simulink model "xb_fft_32pt_core"  (Simulink 7.8)
settings: Solver=ode45  StartTime=0.0  StopTime=10.0  RelTol=1e-3
libraries: xbsIndex_r4 x1517, xbsReplacements_r4 x12
(part 1 of 9)
settings Model: Creator=dan  LastModifiedBy=dan
settings DebuggingCC: FcnCallInpInsideContextMsg=Use local settings  StrictBusMsg=Warning

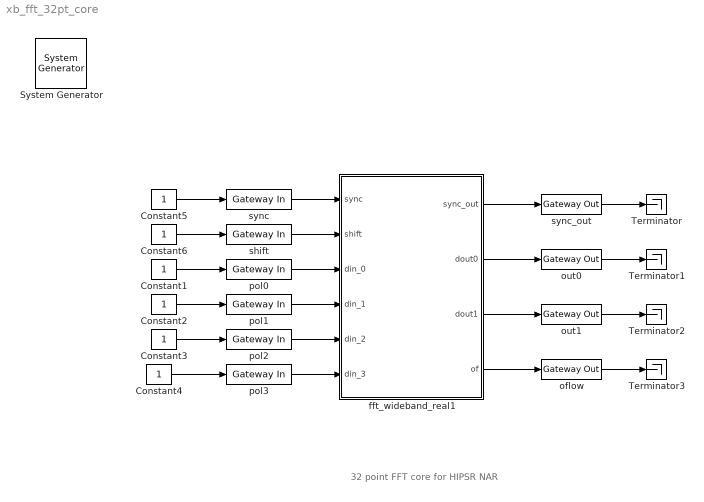
== system xb_fft_32pt_core ==
  note: 32 point FFT core for HIPSR NAR
  " System Generator" : xbsIndex_r4/ System Generator  Tag=genX  xilinxfamily=virtex5  part=xc5vsx95t  speed=-2  package=ff1136  synthesis_tool=XST  clock_wrapper=Clock Enables  directory=/designs/dan/13.x/designs/old/noise_diode/bb/xb_fft_32pt_core  proj_type=Project Navigator  Synth_file=XST Defaults  Impl_file=ISE Defaults  testbench=off  simulink_period=1  sysclk_period=10  dcm_input_clock_period=10  incr_netlist=off  trim_vbits=Everywhere in SubSystem  dbl_ovrd=According to Block Masks  core_generation=According to Block Masks  run_coregen=off  deprecated_control=off  eval_field=0  block_type=sysgen
      settings: block_version=11.4
  Constant{1..6} (6 alike) : Constant
  Terminator{,1..3} (4 alike) : Terminator
  fft_wideband_real1 : Subsystem  AncestorBlock=xblocks_library_ffts/fft_wideband_real  mask(fft_wideband_real){FFTSize=5, n_inputs=2, input_bit_width=18, coeff_bit_width=18, unscramble=on, add_latency=2, mult_latency=3, bram_latency=2, conv_latency=1, input_latency=0, biplex_direct_latency=0, quantization=Truncate, overflow=Wrap, arch=Virtex5, opt_target=logic, coeffs_bit_limit=11, delays_bit_limit=11, specify_mult=on, mult_spec=ones(1,5), hardcode_shifts=on, shift_schedule=ones(1,5), dsp48_adders=on, bit_growth_chart=[0], negate_latency=3, negate_dsp48e=on}
      mask prompts: FFTSize "Size of FFT: (2^? pts)"; n_inputs "Number of Simultaneous Inputs: (2^?)"; input_bit_width "Input Bit Width"; coeff_bit_width "Coefficient Bit Width"; unscramble "Unscramble output (ie, put channels in canonical order)"; add_latency "Add Latency"; mult_latency "Mult Latency"; bram_latency "BRAM Latency"; conv_latency "Convert Latency"; input_latency "Input Latency"; biplex_direct_latency "Latency between biplexes and fft_direct"; quantization "Quantization Behavior"; overflow "Overflow Behavior"; arch "Architecture"; opt_target "Use less"; coeffs_bit_limit "Number bits above which to store stage's coefficients in BRAM (2^? bits)"; delays_bit_limit "Number bits above which to store stage's delays in BRAM (2^? bits)"; specify_mult "Specify multiplier use (behavioral HDL if not specified)"; mult_spec "Multiplier specification (0=core, 1=embedded, 2=behavioural) (left=1st stage)"; hardcode_shifts "Hardcode shift schedule"; shift_schedule "Shift schedule"; dsp48_adders "DSP48 adders in butterfly"; bit_growth_chart "Bit growth vector"; negate_latency "Negate latency"; negate_dsp48e "Negate with DSP48E"
      mask help:
      | A real-sampled wideband FFT.
      |
      | (xBlock version)
      mask init:
      | config.source = str2func('fft_wideband_real_init_xblock');
      | config.toplevel = gcb;
      | config.depend = get_dependlist('fft_wideband_real');
      | set_param(gcb,'LinkStatus','inactive');
      | xBlock(config, {config.toplevel, ...
      |    'FFTSize', FFTSize, ...
      |    'n_inputs', n_inputs, ...
      |    'input_bit_width', input_bit_width, ...
      |    'coeff_bit_width', coeff_bit_width, ...
      |    'unscramble', unscramble, ...
      |    'add_latency', add_latency, ...
      |    'mult_latency', mult_latency, ...
      |    'bram_latency', bram_latency, ...
      |    'conv_latency', conv_latency, ...
      |    'input_latency', input_latency, ...
      |    'biplex_direct_latency', biplex_direct_latency, ...
      |    'quantization', quantization, ...
      |    'overflow', overflow, ...
      |    'arch', arch, ...
      |    'opt_target', opt_target, ...
      |    'coeffs_bit_limit', coeffs_bit_limit, ...
      |    'delays_bit_limit', delays_bit_limit, ...    
      |    'specify_mult', specify_mult, ...
      |    'mult_spec', mult_spec, ...
      |    'hardcode_shifts', hardcode_shifts, ...
      |    'shift_schedule', shift_schedule, ...
      |    'dsp48_adders', dsp48_adders, ...
      |    'bit_growth_chart', bit_growth_chart, ....
      |    'negate_latency', negate_latency, ...
      |    'negate_dsp48e', negate_dsp48e, ...
      | });
      settings: CopyFcn=fft_wideband_real_init(gcb);
      settings: AttributesFormatString=|
      | 5 stages
      | (18,18)
      | Truncate
      | Wrap
      | 0 0 0 0 0 0
      mask Help: eval('xlWeb(''http://casper.berkeley.edu/wiki/Fft_wideband_real'')')
      mask StyleString: edit,edit,edit,edit,checkbox,edit,edit,edit,edit,edit,edit,popup(Truncate|Round  (unbiased: +/- Inf)|Round  (unbiased: Even Values)),popup(Wrap|Saturate|Error),popup(Virtex2Pro|Virtex5),popup(logic|multipliers),edit,edit,checkbox,edit,checkbox,edit,checkbox,edit,edit,checkbox
      mask CallbackString:
      | bit_growth_chart = eval(get_param(gcb,'bit_growth_chart'));
      | FFTSize = eval(get_param(gcb,'FFTSize'));
      | bit_growth_chart = [reshape(bit_growth_chart, 1, []) zeros(1,FFTSize)];
      | bit_growth_sum = sum(bit_growth_chart(1:FFTSize));
      | input_bit_width = eval(get_param(gcb,'input_bit_width'));
      | if input_bit_width + bit_growth_sum > 18
      |     disp('Total bit width cannot exceed 18. Forcing to 0 bit growth');
      |     set_param(gcb,'bit_growth_chart','[0]');
      | end||bit_growth_chart = eval(get_param(gcb,'bit_growth_chart'));
      | FFTSize = eval(get_param(gcb,'FFTSize'));
      | bit_growth_chart = [reshape(bit_growth_chart, 1, []) zeros(1,FFTSize)];
      | bit_growth_sum = sum(bit_growth_chart(1:FFTSize));
      | input_bit_width = eval(get_param(gcb,'input_bit_width'));
      | if input_bit_width + bit_growth_sum > 18
      |     disp('Total bit width cannot exceed 18. Forcing to 0 bit growth');
      |     set_param(gcb,'bit_growth_chart','[0]');
      | end|||||||||||fft_callback_arch(gcb);||||specify_mult = get_param(gcb, 'specify_mult');
      | set_param_state(gcb, 'mult_spec', specify_mult);||hardcode_shifts = get_param(gcb, 'hardcode_shifts');
      | set_param_state(gcb, 'shift_schedule', hardcode_shifts);||fft_callback_dsp48_adders(gcb);|bit_growth_chart = eval(get_param(gcb,'bit_growth_chart'));
      | FFTSize = eval(get_param(gcb,'FFTSize'));
      | bit_growth_chart = [reshape(bit_growth_chart, 1, []) zeros(1,FFTSize)];
      | bit_growth_sum = sum(bit_growth_chart(1:FFTSize));
      | input_bit_width = eval(get_param(gcb,'input_bit_width'));
      | if input_bit_width + bit_growth_sum > 18
      |     disp('Total bit width cannot exceed 18. Forcing to 0 bit growth');
      |     set_param(gcb,'bit_growth_chart','[0]');
      | end||
      mask TabNameString: Basic,Basic,Basic,Basic,Basic,Latency,Latency,Latency,Latency,Latency,Latency,Implementation,Implementation,Implementation,Implementation,Implementation,Implementation,Implementation,Implementation,Implementation,Implementation,Implementation,Basic,Basic,Basic
  oflow : xbsIndex_r4/Gateway Out  inherit_from_input=off  hdl_port=on  timing_constraint=None  locs_specified=off  LOCs={}  UseAsDAC=off  DACChannel='1'  block_type=gatewayout
      settings: infoedit="Gateway out block.  Converts Xilinx fixed point inputs into ouputs of type Simulink integer, double, or fixed point.<br><br>Hardware notes:  In hardware these blocks become top level output ports or are discarded, depending on how they are configured."  block_version=11.4
  out0 : xbsIndex_r4/Gateway Out  inherit_from_input=off  hdl_port=on  timing_constraint=None  locs_specified=off  LOCs={}  UseAsDAC=off  DACChannel='1'  block_type=gatewayout
      settings: infoedit="Gateway out block.  Converts Xilinx fixed point inputs into ouputs of type Simulink integer, double, or fixed point.<br><br>Hardware notes:  In hardware these blocks become top level output ports or are discarded, depending on how they are configured."  block_version=11.4
  out1 : xbsIndex_r4/Gateway Out  inherit_from_input=off  hdl_port=on  timing_constraint=None  locs_specified=off  LOCs={}  UseAsDAC=off  DACChannel='1'  block_type=gatewayout
      settings: infoedit="Gateway out block.  Converts Xilinx fixed point inputs into ouputs of type Simulink integer, double, or fixed point.<br><br>Hardware notes:  In hardware these blocks become top level output ports or are discarded, depending on how they are configured."  block_version=11.4
  pol{0..3} (4 alike) : xbsIndex_r4/Gateway In  gui_display_data_type=Fixed-point  arith_type="Signed  (2's comp)"  n_bits=18  bin_pt=17  preci_type=Single  exp_width=8  frac_width=24  quantization="Round  (unbiased: +/- Inf)"  overflow=Saturate  period=1  dbl_ovrd=off  timing_constraint=None  locs_specified=off  LOCs={}  inherit_from_input=off  UseAsADC=off  ADCChannel='1'  hdl_port=on  block_type=gatewayin
      settings: infoedit="Gateway in block.  Converts inputs of type Simulink integer, double and fixed point to  Xilinx fixed point type.<br><br>Hardware notes:  In hardware these blocks become top level input ports."  block_version=11.4
  shift : xbsIndex_r4/Gateway In  gui_display_data_type=Fixed-point  arith_type=Unsigned  n_bits=32  bin_pt=0  preci_type=Single  exp_width=8  frac_width=24  quantization="Round  (unbiased: +/- Inf)"  overflow=Saturate  period=1  dbl_ovrd=off  timing_constraint=None  locs_specified=off  LOCs={}  inherit_from_input=off  UseAsADC=off  ADCChannel='1'  hdl_port=on  block_type=gatewayin
      settings: infoedit="Gateway in block.  Converts inputs of type Simulink integer, double and fixed point to  Xilinx fixed point type.<br><br>Hardware notes:  In hardware these blocks become top level input ports."  block_version=11.4
  sync : xbsIndex_r4/Gateway In  gui_display_data_type=Fixed-point  arith_type=Boolean  n_bits=16  bin_pt=14  preci_type=Single  exp_width=8  frac_width=24  quantization="Round  (unbiased: +/- Inf)"  overflow=Saturate  period=1  dbl_ovrd=off  timing_constraint=None  locs_specified=off  LOCs={}  inherit_from_input=off  UseAsADC=off  ADCChannel='1'  hdl_port=on  block_type=gatewayin
      settings: infoedit="Gateway in block.  Converts inputs of type Simulink integer, double and fixed point to  Xilinx fixed point type.<br><br>Hardware notes:  In hardware these blocks become top level input ports."  block_version=11.4
  sync_out : xbsIndex_r4/Gateway Out  inherit_from_input=off  hdl_port=on  timing_constraint=None  locs_specified=off  LOCs={}  UseAsDAC=off  DACChannel='1'  block_type=gatewayout
      settings: infoedit="Gateway out block.  Converts Xilinx fixed point inputs into ouputs of type Simulink integer, double, or fixed point.<br><br>Hardware notes:  In hardware these blocks become top level output ports or are discarded, depending on how they are configured."  block_version=11.4
  wires:
  Constant5/1 -> sync/1
  Constant1/1 -> pol0/1
  Constant4/1 -> pol3/1
  Constant3/1 -> pol2/1
  Constant2/1 -> pol1/1
  Constant6/1 -> shift/1
  fft_wideband_real1/1(sync_out) -> sync_out/1
  fft_wideband_real1/2(dout0) -> out0/1
  fft_wideband_real1/3(dout1) -> out1/1
  fft_wideband_real1/4(of) -> oflow/1
  sync_out/1 -> Terminator/1
  oflow/1 -> Terminator3/1
  out1/1 -> Terminator2/1
  out0/1 -> Terminator1/1
  sync/1 -> fft_wideband_real1/1(sync)
  shift/1 -> fft_wideband_real1/2(shift)
  pol0/1 -> fft_wideband_real1/3(din_0)
  pol1/1 -> fft_wideband_real1/4(din_1)
  pol2/1 -> fft_wideband_real1/5(din_2)
  pol3/1 -> fft_wideband_real1/6(din_3)

== system xb_fft_32pt_core/fft_wideband_real1 ==
  sync : Inport
  shift : Inport  Port=2
  din_0 : Inport  Port=3
  din_1 : Inport  Port=4
  din_2 : Inport  Port=5
  din_3 : Inport  Port=6
  fft_biplex_real_4x0 : Subsystem
      settings: AttributesFormatString=|
      | Virtex5
      | 3 stages
      | [18,18]
      | Truncate
      | Wrap
      | 0 0 0 0 0 0 0 0 0
  fft_direct : Subsystem
      settings: AttributesFormatString=|
      | Virtex5
      | stages [4  5] of 5
      | [18,18]
      | Truncate
      | Wrap
      | 0 0 0 0 0
  fft_unscrambler : Subsystem
      settings: AttributesFormatString=FFTSize=4, n_inputs=1
  in_del_4x0pol1 : Subsystem
      settings: AttributesFormatString=Latency = 0
  in_del_4x0pol2 : Subsystem
      settings: AttributesFormatString=Latency = 0
  in_del_4x0pol3 : Subsystem
      settings: AttributesFormatString=Latency = 0
  in_del_4x0pol4 : Subsystem
      settings: AttributesFormatString=Latency = 0
  in_del_sync_4x0 : Subsystem
      settings: AttributesFormatString=Latency = 0
  of_det : xbsIndex_r4/Logical  logical_function=OR  inputs=2  en=off  latency=1  precision=Full  arith_type=Unsigned  n_bits=16  bin_pt=0  align_bp=on  dbl_ovrd=off  block_type=logical
  out_del_4x0pol1 : Subsystem
      settings: AttributesFormatString=Latency = 0
  out_del_4x0pol2 : Subsystem
      settings: AttributesFormatString=Latency = 0
  out_del_4x0pol3 : Subsystem
      settings: AttributesFormatString=Latency = 0
  out_del_4x0pol4 : Subsystem
      settings: AttributesFormatString=Latency = 0
  out_del_sync_4x0 : Subsystem
      settings: AttributesFormatString=Latency = 0
  shift_slice : xbsIndex_r4/Slice  nbits=2  boolean_output=off  mode=Lower Bit Location + Width  bit1=0  base1=MSB of Input  bit0=3  base0=LSB of Input  dbl_ovrd=off  block_type=slice
  sync_out : Outport
  dout0 : Outport  Port=2
  dout1 : Outport  Port=3
  of : Outport  Port=4
  wires:
  shift/1 -> fft_biplex_real_4x0/2(shift), shift_slice/1
  of_det/1 -> of/1
  fft_direct/6(of) -> of_det/2
  fft_biplex_real_4x0/6(of) -> of_det/1
  fft_unscrambler/3(Out2) -> dout1/1
  fft_unscrambler/2(Out1) -> dout0/1
  fft_unscrambler/1(sync_out) -> sync_out/1
  fft_direct/3(dout_1) -> fft_unscrambler/3(In2)
  fft_direct/2(dout_0) -> fft_unscrambler/2(In1)
  fft_direct/1(sync_out) -> fft_unscrambler/1(sync)
  out_del_4x0pol4/1(q) -> fft_direct/6(din_3)
  out_del_4x0pol3/1(q) -> fft_direct/5(din_2)
  out_del_4x0pol2/1(q) -> fft_direct/4(din_1)
  out_del_4x0pol1/1(q) -> fft_direct/3(din_0)
  shift_slice/1 -> fft_direct/2(shift)
  out_del_sync_4x0/1(q) -> fft_direct/1(sync)
  fft_biplex_real_4x0/1(sync_out) -> out_del_sync_4x0/1(d)
  fft_biplex_real_4x0/5(pol4_out) -> out_del_4x0pol4/1(d)
  fft_biplex_real_4x0/4(pol3_out) -> out_del_4x0pol3/1(d)
  fft_biplex_real_4x0/3(pol2_out) -> out_del_4x0pol2/1(d)
  fft_biplex_real_4x0/2(pol1_out) -> out_del_4x0pol1/1(d)
  in_del_4x0pol4/1(q) -> fft_biplex_real_4x0/6(pol4)
  in_del_4x0pol3/1(q) -> fft_biplex_real_4x0/5(pol3)
  in_del_4x0pol2/1(q) -> fft_biplex_real_4x0/4(pol2)
  in_del_4x0pol1/1(q) -> fft_biplex_real_4x0/3(pol1)
  in_del_sync_4x0/1(q) -> fft_biplex_real_4x0/1(sync)
  din_3/1 -> in_del_4x0pol4/1(d)
  din_2/1 -> in_del_4x0pol3/1(d)
  din_1/1 -> in_del_4x0pol2/1(d)
  din_0/1 -> in_del_4x0pol1/1(d)
  sync/1 -> in_del_sync_4x0/1(d)

== system xb_fft_32pt_core/fft_wideband_real1/fft_biplex_real_4x0 ==
  sync : Inport
  shift : Inport  Port=2
  pol1 : Inport  Port=3
  pol2 : Inport  Port=4
  pol3 : Inport  Port=5
  pol4 : Inport  Port=6
  bi_real_unscr_4x : Subsystem
  biplex_core : Subsystem
      settings: AttributesFormatString=|
      | 3 stages
      | reduce logic
      | Virtex5
  ri_to_c_pol1 : Subsystem
  ri_to_c_pol2 : Subsystem
  sync_out : Outport
  pol1_out : Outport  Port=2
  pol2_out : Outport  Port=3
  pol3_out : Outport  Port=4
  pol4_out : Outport  Port=5
  of : Outport  Port=6
  wires:
  bi_real_unscr_4x/5(pol4_out) -> pol4_out/1
  bi_real_unscr_4x/4(pol3_out) -> pol3_out/1
  bi_real_unscr_4x/3(pol2_out) -> pol2_out/1
  bi_real_unscr_4x/2(pol1_out) -> pol1_out/1
  bi_real_unscr_4x/1(sync_out) -> sync_out/1
  biplex_core/3(out2) -> bi_real_unscr_4x/3(odd)
  biplex_core/2(out1) -> bi_real_unscr_4x/2(even)
  biplex_core/1(sync_out) -> bi_real_unscr_4x/1(sync)
  biplex_core/4(of) -> of/1
  ri_to_c_pol2/1(c) -> biplex_core/4(pol2)
  ri_to_c_pol1/1(c) -> biplex_core/3(pol1)
  shift/1 -> biplex_core/2(shift)
  sync/1 -> biplex_core/1(sync)
  pol4/1 -> ri_to_c_pol2/2(im)
  pol3/1 -> ri_to_c_pol2/1(re)
  pol2/1 -> ri_to_c_pol1/2(im)
  pol1/1 -> ri_to_c_pol1/1(re)

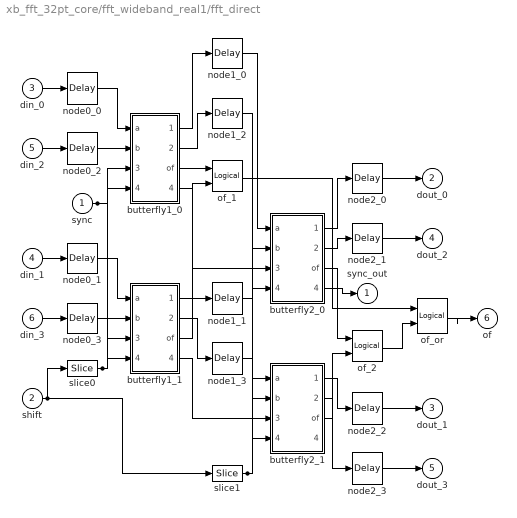
== system xb_fft_32pt_core/fft_wideband_real1/fft_direct ==
  sync : Inport
  shift : Inport  Port=2
  din_0 : Inport  Port=3
  din_1 : Inport  Port=4
  din_2 : Inport  Port=5
  din_3 : Inport  Port=6
  butterfly1_0 : Subsystem
      settings: AttributesFormatString=|
      | twiddle_general_4mult
      | coeffs in slices
      | Bit growth:0
  butterfly1_1 : Subsystem
      settings: AttributesFormatString=|
      | twiddle_general_4mult
      | coeffs in slices
      | Bit growth:0
  butterfly2_0 : Subsystem
      settings: AttributesFormatString=|
      | twiddle_general_4mult
      | coeffs in slices
      | Bit growth:0
  butterfly2_1 : Subsystem
      settings: AttributesFormatString=|
      | twiddle_general_4mult
      | coeffs in slices
      | Bit growth:0
  node0_{0..3} (4 alike) : xbsIndex_r4/Delay  rst=off  infoeditControl=Selection of Reset will increase slice count due to use of real FFs and instead of SRLs  en=off  latency=0  dbl_ovrd=off  reg_retiming=off  block_type=delay
  node1_{0..3} (4 alike) : xbsIndex_r4/Delay  rst=off  infoeditControl=Selection of Reset will increase slice count due to use of real FFs and instead of SRLs  en=off  latency=0  dbl_ovrd=off  reg_retiming=off  block_type=delay
  node2_{0..3} (4 alike) : xbsIndex_r4/Delay  rst=off  infoeditControl=Selection of Reset will increase slice count due to use of real FFs and instead of SRLs  en=off  latency=0  dbl_ovrd=off  reg_retiming=off  block_type=delay
  of_1 : xbsIndex_r4/Logical  logical_function=OR  inputs=2  en=off  latency=1  precision=Full  arith_type=Unsigned  n_bits=16  bin_pt=0  align_bp=on  dbl_ovrd=off  block_type=logical
  of_2 : xbsIndex_r4/Logical  logical_function=OR  inputs=2  en=off  latency=1  precision=Full  arith_type=Unsigned  n_bits=16  bin_pt=0  align_bp=on  dbl_ovrd=off  block_type=logical
  of_or : xbsIndex_r4/Logical  logical_function=OR  inputs=2  en=off  latency=0  precision=Full  arith_type=Unsigned  n_bits=16  bin_pt=0  align_bp=on  dbl_ovrd=off  block_type=logical
  slice0 : xbsIndex_r4/Slice  nbits=1  boolean_output=on  mode=Lower Bit Location + Width  bit1=0  base1=MSB of Input  bit0=0  base0=LSB of Input  dbl_ovrd=off  block_type=slice
  slice1 : xbsIndex_r4/Slice  nbits=1  boolean_output=on  mode=Lower Bit Location + Width  bit1=0  base1=MSB of Input  bit0=1  base0=LSB of Input  dbl_ovrd=off  block_type=slice
  sync_out : Outport
  dout_0 : Outport  Port=2
  dout_1 : Outport  Port=3
  dout_2 : Outport  Port=4
  dout_3 : Outport  Port=5
  of : Outport  Port=6
  wires:
  shift/1 -> slice1/1, slice0/1
  sync/1 -> butterfly1_1/3(sync), butterfly1_0/3(sync)
  slice0/1 -> butterfly1_1/4(shift), butterfly1_0/4(shift)
  slice1/1 -> butterfly2_1/4(shift), butterfly2_0/4(shift)
  butterfly2_0/4(sync_out) -> sync_out/1
  of_or/1 -> of/1
  of_2/1 -> of_or/2
  of_1/1 -> of_or/1
  butterfly2_1/3(of) -> of_2/2
  butterfly2_0/3(of) -> of_2/1
  butterfly2_1/2(a-bw) -> node2_3/1
  butterfly2_1/1(a+bw) -> node2_2/1
  butterfly1_1/4(sync_out) -> butterfly2_1/3(sync)
  node1_3/1 -> butterfly2_1/2(b)
  node1_2/1 -> butterfly2_1/1(a)
  butterfly2_0/2(a-bw) -> node2_1/1
  butterfly2_0/1(a+bw) -> node2_0/1
  butterfly1_0/4(sync_out) -> butterfly2_0/3(sync)
  node1_1/1 -> butterfly2_0/2(b)
  node1_0/1 -> butterfly2_0/1(a)
  butterfly1_1/3(of) -> of_1/2
  butterfly1_0/3(of) -> of_1/1
  butterfly1_1/2(a-bw) -> node1_3/1
  butterfly1_1/1(a+bw) -> node1_1/1
  node0_3/1 -> butterfly1_1/2(b)
  node0_1/1 -> butterfly1_1/1(a)
  butterfly1_0/2(a-bw) -> node1_2/1
  butterfly1_0/1(a+bw) -> node1_0/1
  node0_2/1 -> butterfly1_0/2(b)
  node0_0/1 -> butterfly1_0/1(a)
  node2_3/1 -> dout_3/1
  node2_2/1 -> dout_1/1
  node2_1/1 -> dout_2/1
  node2_0/1 -> dout_0/1
  din_3/1 -> node0_3/1
  din_2/1 -> node0_2/1
  din_1/1 -> node0_1/1
  din_0/1 -> node0_0/1

== system xb_fft_32pt_core/fft_wideband_real1/fft_unscrambler ==
  sync : Inport
  In1 : Inport  Port=2
  In2 : Inport  Port=3
  const : xbsIndex_r4/Constant  const=1  gui_display_data_type=Fixed-point  arith_type=Boolean  n_bits=1  bin_pt=0  preci_type=Single  exp_width=8  frac_width=24  explicit_period=on  period=1  equ=P=C  opselect=C  inp2=PCIN>>17  opr=+  inp1=P  carry=CIN  dbl_ovrd=off  block_type=constant
  reorder1 : Subsystem
      settings: AttributesFormatString=order=3
  square_transposer1 : Subsystem
      settings: AttributesFormatString=n_inputs=1
  sync_out : Outport
  Out1 : Outport  Port=2
  Out2 : Outport  Port=3
  wires:
  square_transposer1/3(Out2) -> reorder1/4(din1)  "xlsub2_reorder_In2"
  square_transposer1/2(Out1) -> reorder1/3(din0)  "xlsub2_reorder_In1"
  square_transposer1/1(sync_out) -> reorder1/1(sync)
  In2/1 -> square_transposer1/3(In2)
  In1/1 -> square_transposer1/2(In1)
  sync/1 -> square_transposer1/1(sync)
  reorder1/4(dout1) -> Out2/1
  reorder1/3(dout0) -> Out1/1
  reorder1/1(sync_out) -> sync_out/1
  const/1 -> reorder1/2(en)

== system xb_fft_32pt_core/fft_wideband_real1/in_del_4x0pol1 ==
  d : Inport
  q : Outport
  wires:
  d/1 -> q/1

== system xb_fft_32pt_core/fft_wideband_real1/in_del_4x0pol2 ==
  d : Inport
  q : Outport
  wires:
  d/1 -> q/1

== system xb_fft_32pt_core/fft_wideband_real1/in_del_4x0pol3 ==
  d : Inport
  q : Outport
  wires:
  d/1 -> q/1

== system xb_fft_32pt_core/fft_wideband_real1/in_del_4x0pol4 ==
  d : Inport
  q : Outport
  wires:
  d/1 -> q/1

== system xb_fft_32pt_core/fft_wideband_real1/in_del_sync_4x0 ==
  d : Inport
  q : Outport
  wires:
  d/1 -> q/1

== system xb_fft_32pt_core/fft_wideband_real1/out_del_4x0pol1 ==
  d : Inport
  q : Outport
  wires:
  d/1 -> q/1

== system xb_fft_32pt_core/fft_wideband_real1/out_del_4x0pol2 ==
  d : Inport
  q : Outport
  wires:
  d/1 -> q/1

== system xb_fft_32pt_core/fft_wideband_real1/out_del_4x0pol3 ==
  d : Inport
  q : Outport
  wires:
  d/1 -> q/1

== system xb_fft_32pt_core/fft_wideband_real1/out_del_4x0pol4 ==
  d : Inport
  q : Outport
  wires:
  d/1 -> q/1

== system xb_fft_32pt_core/fft_wideband_real1/out_del_sync_4x0 ==
  d : Inport
  q : Outport
  wires:
  d/1 -> q/1

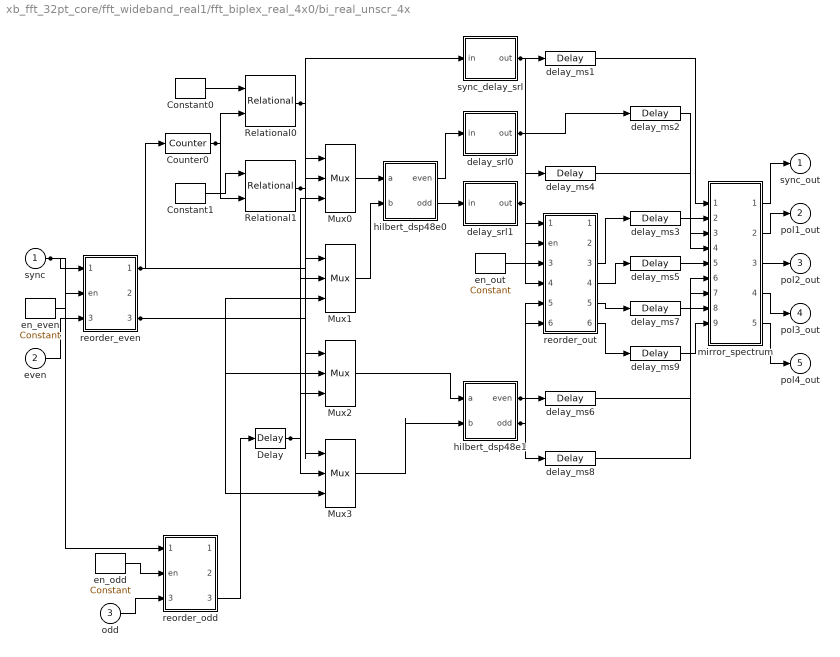
== system xb_fft_32pt_core/fft_wideband_real1/fft_biplex_real_4x0/bi_real_unscr_4x ==
  sync : Inport
  even : Inport  Port=2
  odd : Inport  Port=3
  Constant0 : xbsIndex_r4/Constant  const=3  gui_display_data_type=Fixed-point  arith_type=Unsigned  n_bits=3  bin_pt=0  preci_type=Single  exp_width=8  frac_width=24  explicit_period=on  period=1  equ=P=C  opselect=C  inp2=PCIN>>17  opr=+  inp1=P  carry=CIN  dbl_ovrd=off  block_type=constant
  Constant1 : xbsIndex_r4/Constant  const=7  gui_display_data_type=Fixed-point  arith_type=Unsigned  n_bits=3  bin_pt=0  preci_type=Single  exp_width=8  frac_width=24  explicit_period=on  period=1  equ=P=C  opselect=C  inp2=PCIN>>17  opr=+  inp1=P  carry=CIN  dbl_ovrd=off  block_type=constant
  Counter0 : xbsIndex_r4/Counter  cnt_type=Free Running  cnt_to=Inf  operation=Up  start_count=0  cnt_by_val=1  arith_type=Unsigned  n_bits=3  bin_pt=0  load_pin=off  rst=on  en=off  explicit_period=on  period=1  dbl_ovrd=off  use_behavioral_HDL=off  implementation=Fabric  block_type=counter
  Delay : xbsIndex_r4/Delay  rst=off  infoeditControl=Selection of Reset will increase slice count due to use of real FFs and instead of SRLs  en=off  latency=1  dbl_ovrd=off  reg_retiming=off  block_type=delay
  Mux{0..3} (4 alike) : xbsIndex_r4/Mux  inputs=2  en=off  latency=1  precision=Full  arith_type=Unsigned  n_bits=16  bin_pt=14  quantization=Truncate  overflow=Wrap  dbl_ovrd=off  block_type=mux
  Relational0 : xbsIndex_r4/Relational  mode=a=b  en=off  latency=1  dbl_ovrd=off  block_type=relational
  Relational1 : xbsIndex_r4/Relational  mode=a=b  en=off  latency=1  dbl_ovrd=off  block_type=relational
  delay_ms{1..9} (9 alike) : xbsIndex_r4/Delay  rst=off  infoeditControl=Selection of Reset will increase slice count due to use of real FFs and instead of SRLs  en=off  latency=1  dbl_ovrd=off  reg_retiming=off  block_type=delay
  delay_srl0 : Subsystem
  delay_srl1 : Subsystem
  en_even : xbsIndex_r4/Constant  const=1  gui_display_data_type=Fixed-point  arith_type=Boolean  n_bits=1  bin_pt=0  preci_type=Single  exp_width=8  frac_width=24  explicit_period=on  period=1  equ=P=C  opselect=C  inp2=PCIN>>17  opr=+  inp1=P  carry=CIN  dbl_ovrd=off  block_type=constant
  en_odd : xbsIndex_r4/Constant  const=1  gui_display_data_type=Fixed-point  arith_type=Boolean  n_bits=1  bin_pt=0  preci_type=Single  exp_width=8  frac_width=24  explicit_period=on  period=1  equ=P=C  opselect=C  inp2=PCIN>>17  opr=+  inp1=P  carry=CIN  dbl_ovrd=off  block_type=constant
  en_out : xbsIndex_r4/Constant  const=1  gui_display_data_type=Fixed-point  arith_type=Boolean  n_bits=1  bin_pt=0  preci_type=Single  exp_width=8  frac_width=24  explicit_period=on  period=1  equ=P=C  opselect=C  inp2=PCIN>>17  opr=+  inp1=P  carry=CIN  dbl_ovrd=off  block_type=constant
  hilbert_dsp48e0 : Subsystem
  hilbert_dsp48e1 : Subsystem
  mirror_spectrum : Subsystem
  reorder_even : Subsystem
      settings: AttributesFormatString=order=2
  reorder_odd : Subsystem
      settings: AttributesFormatString=order=2
  reorder_out : Subsystem
      settings: AttributesFormatString=order=2
  sync_delay_srl : Subsystem
  sync_out : Outport
  pol1_out : Outport  Port=2
  pol2_out : Outport  Port=3
  pol3_out : Outport  Port=4
  pol4_out : Outport  Port=5
  wires:
  sync/1 -> reorder_odd/1(sync), reorder_even/1(sync)
  reorder_even/1(sync_out) -> sync_delay_srl/1(in), Counter0/1
  Counter0/1 -> Relational1/2, Relational0/2
  Relational0/1 -> Mux3/1, Mux0/1
  reorder_even/3(dout0) -> Mux3/3, Mux2/2, Mux1/3, Mux0/2
  Delay/1 -> Mux3/2, Mux2/3, Mux1/2, Mux0/3
  Relational1/1 -> Mux2/1, Mux1/1
  sync_delay_srl/1(out) -> delay_ms1/1, reorder_out/1(sync)
  delay_srl0/1(out) -> delay_ms2/1, reorder_out/3(din0)
  delay_srl1/1(out) -> delay_ms4/1, reorder_out/4(din1)
  hilbert_dsp48e1/1(even) -> delay_ms6/1, reorder_out/5(din2)
  hilbert_dsp48e1/2(odd) -> delay_ms8/1, reorder_out/6(din3)
  mirror_spectrum/5(dout3) -> pol4_out/1
  mirror_spectrum/4(dout2) -> pol3_out/1
  mirror_spectrum/3(dout1) -> pol2_out/1
  mirror_spectrum/2(dout0) -> pol1_out/1
  mirror_spectrum/1(sync_out) -> sync_out/1
  delay_ms9/1 -> mirror_spectrum/9(reo_in3)
  delay_ms8/1 -> mirror_spectrum/8(din3)
  delay_ms7/1 -> mirror_spectrum/7(reo_in2)
  delay_ms6/1 -> mirror_spectrum/6(din2)
  delay_ms5/1 -> mirror_spectrum/5(reo_in1)
  delay_ms4/1 -> mirror_spectrum/4(din1)
  delay_ms3/1 -> mirror_spectrum/3(reo_in0)
  delay_ms2/1 -> mirror_spectrum/2(din0)
  delay_ms1/1 -> mirror_spectrum/1(sync)
  reorder_out/6(dout3) -> delay_ms9/1
  reorder_out/5(dout2) -> delay_ms7/1
  reorder_out/4(dout1) -> delay_ms5/1
  reorder_out/3(dout0) -> delay_ms3/1
  en_out/1 -> reorder_out/2(en)
  hilbert_dsp48e0/2(odd) -> delay_srl1/1(in)
  hilbert_dsp48e0/1(even) -> delay_srl0/1(in)
  Mux3/1 -> hilbert_dsp48e1/2(b)
  Mux2/1 -> hilbert_dsp48e1/1(a)
  Mux1/1 -> hilbert_dsp48e0/2(b)
  Mux0/1 -> hilbert_dsp48e0/1(a)
  reorder_odd/3(dout0) -> Delay/1
  Constant1/1 -> Relational1/1
  Constant0/1 -> Relational0/1
  odd/1 -> reorder_odd/3(din0)
  en_odd/1 -> reorder_odd/2(en)
  even/1 -> reorder_even/3(din0)
  en_even/1 -> reorder_even/2(en)

== system xb_fft_32pt_core/fft_wideband_real1/fft_biplex_real_4x0/biplex_core ==
  sync : Inport
  shift : Inport  Port=2
  pol1 : Inport  Port=3
  pol2 : Inport  Port=4
  Constant : xbsIndex_r4/Constant  const=0  gui_display_data_type=Fixed-point  arith_type=Boolean  n_bits=16  bin_pt=14  preci_type=Single  exp_width=8  frac_width=24  explicit_period=off  period=1  equ=P=C  opselect=C  inp2=PCIN>>17  opr=+  inp1=P  carry=CIN  dbl_ovrd=off  block_type=constant
  Slice1 : xbsIndex_r4/Slice  nbits=1  boolean_output=off  mode=Upper Bit Location + Width  bit1=-0  base1=MSB of Input  bit0=0  base0=LSB of Input  dbl_ovrd=off  block_type=slice
  Slice2 : xbsIndex_r4/Slice  nbits=1  boolean_output=off  mode=Upper Bit Location + Width  bit1=-0  base1=MSB of Input  bit0=0  base0=LSB of Input  dbl_ovrd=off  block_type=slice
  Slice3 : xbsIndex_r4/Slice  nbits=1  boolean_output=off  mode=Upper Bit Location + Width  bit1=-0  base1=MSB of Input  bit0=0  base0=LSB of Input  dbl_ovrd=off  block_type=slice
  biplex_sel_counter : xbsIndex_r4/Counter  cnt_type=Free Running  cnt_to=Inf  operation=Up  start_count=0  cnt_by_val=1  arith_type=Unsigned  n_bits=3  bin_pt=0  load_pin=off  rst=on  en=off  explicit_period=off  period=1  dbl_ovrd=off  use_behavioral_HDL=off  implementation=Fabric  use_rpm=off  block_type=counter
  fft_stage_1 : Subsystem
      settings: AttributesFormatString=|
      | [1/3]
      | delays in slices
      | coeffs in slices
      | Bit growth = 0
  fft_stage_2 : Subsystem
      settings: AttributesFormatString=|
      | [2/3]
      | delays in slices
      | coeffs in slices
      | Bit growth = 0
  fft_stage_3 : Subsystem
      settings: AttributesFormatString=|
      | [3/3]
      | delays in slices
      | coeffs in slices
      | Bit growth = 0
  stage_2_cnt : xbsIndex_r4/Counter  cnt_type=Free Running  cnt_to=Inf  operation=Up  start_count=0  cnt_by_val=1  arith_type=Unsigned  n_bits=2  bin_pt=0  load_pin=off  rst=on  en=off  explicit_period=off  period=1  dbl_ovrd=off  use_behavioral_HDL=off  implementation=Fabric  use_rpm=off  block_type=counter
  stage_3_cnt : xbsIndex_r4/Counter  cnt_type=Free Running  cnt_to=Inf  operation=Up  start_count=0  cnt_by_val=1  arith_type=Unsigned  n_bits=1  bin_pt=0  load_pin=off  rst=on  en=off  explicit_period=off  period=1  dbl_ovrd=off  use_behavioral_HDL=off  implementation=Fabric  use_rpm=off  block_type=counter
  sync_out : Outport
  out1 : Outport  Port=2
  out2 : Outport  Port=3
  of : Outport  Port=4
  wires:
  sync/1 -> fft_stage_1/4(sync), biplex_sel_counter/1
  shift/1 -> fft_stage_3/5(shift), fft_stage_2/5(shift), fft_stage_1/5(shift)
  fft_stage_1/4(sync_out) -> fft_stage_2/4(sync), stage_2_cnt/1
  fft_stage_2/4(sync_out) -> fft_stage_3/4(sync), stage_3_cnt/1
  fft_stage_3/4(sync_out) -> sync_out/1
  fft_stage_3/3(of) -> of/1
  fft_stage_3/2(out2) -> out2/1
  fft_stage_3/1(out1) -> out1/1
  Slice3/1 -> fft_stage_3/6(biplex_sel)
  fft_stage_2/3(of) -> fft_stage_3/3(of_in)
  fft_stage_2/2(out2) -> fft_stage_3/2(in2)
  fft_stage_2/1(out1) -> fft_stage_3/1(in1)
  stage_3_cnt/1 -> Slice3/1
  Slice2/1 -> fft_stage_2/6(biplex_sel)
  fft_stage_1/3(of) -> fft_stage_2/3(of_in)
  fft_stage_1/2(out2) -> fft_stage_2/2(in2)
  fft_stage_1/1(out1) -> fft_stage_2/1(in1)
  stage_2_cnt/1 -> Slice2/1
  Slice1/1 -> fft_stage_1/6(biplex_sel)
  Constant/1 -> fft_stage_1/3(of_in)
  pol2/1 -> fft_stage_1/2(in2)
  pol1/1 -> fft_stage_1/1(in1)
  biplex_sel_counter/1 -> Slice1/1

== system xb_fft_32pt_core/fft_wideband_real1/fft_biplex_real_4x0/ri_to_c_pol1 ==
  re : Inport
  im : Inport  Port=2
  concat : xbsIndex_r4/Concat  num_inputs=2  dbl_ovrd=off  block_type=concat
  force_im : xbsIndex_r4/Reinterpret  force_arith_type=on  arith_type=Unsigned  force_bin_pt=on  bin_pt=0  block_type=reinterpret
  force_re : xbsIndex_r4/Reinterpret  force_arith_type=on  arith_type=Unsigned  force_bin_pt=on  bin_pt=0  block_type=reinterpret
  c : Outport
  wires:
  force_re/1 -> concat/1
  re/1 -> force_re/1
  force_im/1 -> concat/2
  im/1 -> force_im/1
  concat/1 -> c/1

== system xb_fft_32pt_core/fft_wideband_real1/fft_biplex_real_4x0/ri_to_c_pol2 ==
  re : Inport
  im : Inport  Port=2
  concat : xbsIndex_r4/Concat  num_inputs=2  dbl_ovrd=off  block_type=concat
  force_im : xbsIndex_r4/Reinterpret  force_arith_type=on  arith_type=Unsigned  force_bin_pt=on  bin_pt=0  block_type=reinterpret
  force_re : xbsIndex_r4/Reinterpret  force_arith_type=on  arith_type=Unsigned  force_bin_pt=on  bin_pt=0  block_type=reinterpret
  c : Outport
  wires:
  force_re/1 -> concat/1
  re/1 -> force_re/1
  force_im/1 -> concat/2
  im/1 -> force_im/1
  concat/1 -> c/1

== system xb_fft_32pt_core/fft_wideband_real1/fft_direct/butterfly1_0 ==
  a : Inport
  b : Inport  Port=2
  sync : Inport  Port=3
  shift : Inport  Port=4
  Logical : xbsIndex_r4/Logical  logical_function=OR  inputs=4  en=off  latency=0  precision=Full  arith_type=Unsigned  n_bits=16  bin_pt=0  align_bp=on  dbl_ovrd=off  block_type=logical
  Terminator : Terminator
  arith : Subsystem
  conv_of_1 : Subsystem
      settings: AttributesFormatString=[23,19]->[18,17]
  conv_of_2 : Subsystem
      settings: AttributesFormatString=[23,19]->[18,17]
  conv_of_3 : Subsystem
      settings: AttributesFormatString=[23,19]->[18,17]
  conv_of_4 : Subsystem
      settings: AttributesFormatString=[23,19]->[18,17]
  ri_to_c01 : Subsystem
  ri_to_c23 : Subsystem
  scale_{1..4} (4 alike) : xbsIndex_r4/Scale  scale_factor=-1  dbl_ovrd=off  block_type=scale
  sync_delay : xbsIndex_r4/Delay  rst=off  infoeditControl=Selection of Reset will increase slice count due to use of real FFs and instead of SRLs  en=off  latency=1  dbl_ovrd=off  reg_retiming=on  block_type=delay
  a+bw : Outport
  a-bw : Outport  Port=2
  of : Outport  Port=3
  sync_out : Outport  Port=4
  wires:
  sync_delay/1 -> sync_out/1
  arith/5(sync_out) -> sync_delay/1  "twiddle_sync_out"
  ri_to_c23/1(c) -> a-bw/1
  conv_of_4/1(dout) -> ri_to_c23/2(im)
  conv_of_3/1(dout) -> ri_to_c23/1(re)
  ri_to_c01/1(c) -> a+bw/1
  conv_of_2/1(dout) -> ri_to_c01/2(im)
  conv_of_1/1(dout) -> ri_to_c01/1(re)
  Logical/1 -> of/1
  conv_of_4/2(of) -> Logical/4
  conv_of_3/2(of) -> Logical/3
  conv_of_2/2(of) -> Logical/2
  conv_of_1/2(of) -> Logical/1
  scale_4/1 -> conv_of_4/1(din)
  arith/4(a-bw_im) -> scale_4/1
  scale_3/1 -> conv_of_3/1(din)
  arith/3(a-bw_re) -> scale_3/1
  scale_2/1 -> conv_of_2/1(din)
  arith/2(a+bw_im) -> scale_2/1
  scale_1/1 -> conv_of_1/1(din)
  arith/1(a+bw_re) -> scale_1/1
  shift/1 -> Terminator/1
  sync/1 -> arith/3(sync)
  b/1 -> arith/2(b)
  a/1 -> arith/1(a)

== system xb_fft_32pt_core/fft_wideband_real1/fft_direct/butterfly1_1 ==
  a : Inport
  b : Inport  Port=2
  sync : Inport  Port=3
  shift : Inport  Port=4
  Logical : xbsIndex_r4/Logical  logical_function=OR  inputs=4  en=off  latency=0  precision=Full  arith_type=Unsigned  n_bits=16  bin_pt=0  align_bp=on  dbl_ovrd=off  block_type=logical
  Terminator : Terminator
  arith : Subsystem
  conv_of_1 : Subsystem
      settings: AttributesFormatString=[23,19]->[18,17]
  conv_of_2 : Subsystem
      settings: AttributesFormatString=[23,19]->[18,17]
  conv_of_3 : Subsystem
      settings: AttributesFormatString=[23,19]->[18,17]
  conv_of_4 : Subsystem
      settings: AttributesFormatString=[23,19]->[18,17]
  ri_to_c01 : Subsystem
  ri_to_c23 : Subsystem
  scale_{1..4} (4 alike) : xbsIndex_r4/Scale  scale_factor=-1  dbl_ovrd=off  block_type=scale
  sync_delay : xbsIndex_r4/Delay  rst=off  infoeditControl=Selection of Reset will increase slice count due to use of real FFs and instead of SRLs  en=off  latency=1  dbl_ovrd=off  reg_retiming=on  block_type=delay
  a+bw : Outport
  a-bw : Outport  Port=2
  of : Outport  Port=3
  sync_out : Outport  Port=4
  wires:
  sync_delay/1 -> sync_out/1
  arith/5(sync_out) -> sync_delay/1  "twiddle_sync_out"
  ri_to_c23/1(c) -> a-bw/1
  conv_of_4/1(dout) -> ri_to_c23/2(im)
  conv_of_3/1(dout) -> ri_to_c23/1(re)
  ri_to_c01/1(c) -> a+bw/1
  conv_of_2/1(dout) -> ri_to_c01/2(im)
  conv_of_1/1(dout) -> ri_to_c01/1(re)
  Logical/1 -> of/1
  conv_of_4/2(of) -> Logical/4
  conv_of_3/2(of) -> Logical/3
  conv_of_2/2(of) -> Logical/2
  conv_of_1/2(of) -> Logical/1
  scale_4/1 -> conv_of_4/1(din)
  arith/4(a-bw_im) -> scale_4/1
  scale_3/1 -> conv_of_3/1(din)
  arith/3(a-bw_re) -> scale_3/1
  scale_2/1 -> conv_of_2/1(din)
  arith/2(a+bw_im) -> scale_2/1
  scale_1/1 -> conv_of_1/1(din)
  arith/1(a+bw_re) -> scale_1/1
  shift/1 -> Terminator/1
  sync/1 -> arith/3(sync)
  b/1 -> arith/2(b)
  a/1 -> arith/1(a)

== system xb_fft_32pt_core/fft_wideband_real1/fft_direct/butterfly2_0 ==
  a : Inport
  b : Inport  Port=2
  sync : Inport  Port=3
  shift : Inport  Port=4
  Logical : xbsIndex_r4/Logical  logical_function=OR  inputs=4  en=off  latency=0  precision=Full  arith_type=Unsigned  n_bits=16  bin_pt=0  align_bp=on  dbl_ovrd=off  block_type=logical
  Terminator : Terminator
  arith : Subsystem
  conv_of_1 : Subsystem
      settings: AttributesFormatString=[23,19]->[18,17]
  conv_of_2 : Subsystem
      settings: AttributesFormatString=[23,19]->[18,17]
  conv_of_3 : Subsystem
      settings: AttributesFormatString=[23,19]->[18,17]
  conv_of_4 : Subsystem
      settings: AttributesFormatString=[23,19]->[18,17]
  ri_to_c01 : Subsystem
  ri_to_c23 : Subsystem
  scale_{1..4} (4 alike) : xbsIndex_r4/Scale  scale_factor=-1  dbl_ovrd=off  block_type=scale
  sync_delay : xbsIndex_r4/Delay  rst=off  infoeditControl=Selection of Reset will increase slice count due to use of real FFs and instead of SRLs  en=off  latency=1  dbl_ovrd=off  reg_retiming=on  block_type=delay
  a+bw : Outport
  a-bw : Outport  Port=2
  of : Outport  Port=3
  sync_out : Outport  Port=4
  wires:
  sync_delay/1 -> sync_out/1
  arith/5(sync_out) -> sync_delay/1  "twiddle_sync_out"
  ri_to_c23/1(c) -> a-bw/1
  conv_of_4/1(dout) -> ri_to_c23/2(im)
  conv_of_3/1(dout) -> ri_to_c23/1(re)
  ri_to_c01/1(c) -> a+bw/1
  conv_of_2/1(dout) -> ri_to_c01/2(im)
  conv_of_1/1(dout) -> ri_to_c01/1(re)
  Logical/1 -> of/1
  conv_of_4/2(of) -> Logical/4
  conv_of_3/2(of) -> Logical/3
  conv_of_2/2(of) -> Logical/2
  conv_of_1/2(of) -> Logical/1
  scale_4/1 -> conv_of_4/1(din)
  arith/4(a-bw_im) -> scale_4/1
  scale_3/1 -> conv_of_3/1(din)
  arith/3(a-bw_re) -> scale_3/1
  scale_2/1 -> conv_of_2/1(din)
  arith/2(a+bw_im) -> scale_2/1
  scale_1/1 -> conv_of_1/1(din)
  arith/1(a+bw_re) -> scale_1/1
  shift/1 -> Terminator/1
  sync/1 -> arith/3(sync)
  b/1 -> arith/2(b)
  a/1 -> arith/1(a)

== system xb_fft_32pt_core/fft_wideband_real1/fft_direct/butterfly2_1 ==
  a : Inport
  b : Inport  Port=2
  sync : Inport  Port=3
  shift : Inport  Port=4
  Logical : xbsIndex_r4/Logical  logical_function=OR  inputs=4  en=off  latency=0  precision=Full  arith_type=Unsigned  n_bits=16  bin_pt=0  align_bp=on  dbl_ovrd=off  block_type=logical
  Terminator : Terminator
  arith : Subsystem
  conv_of_1 : Subsystem
      settings: AttributesFormatString=[23,19]->[18,17]
  conv_of_2 : Subsystem
      settings: AttributesFormatString=[23,19]->[18,17]
  conv_of_3 : Subsystem
      settings: AttributesFormatString=[23,19]->[18,17]
  conv_of_4 : Subsystem
      settings: AttributesFormatString=[23,19]->[18,17]
  ri_to_c01 : Subsystem
  ri_to_c23 : Subsystem
  scale_{1..4} (4 alike) : xbsIndex_r4/Scale  scale_factor=-1  dbl_ovrd=off  block_type=scale
  sync_delay : xbsIndex_r4/Delay  rst=off  infoeditControl=Selection of Reset will increase slice count due to use of real FFs and instead of SRLs  en=off  latency=1  dbl_ovrd=off  reg_retiming=on  block_type=delay
  a+bw : Outport
  a-bw : Outport  Port=2
  of : Outport  Port=3
  sync_out : Outport  Port=4
  wires:
  sync_delay/1 -> sync_out/1
  arith/5(sync_out) -> sync_delay/1  "twiddle_sync_out"
  ri_to_c23/1(c) -> a-bw/1
  conv_of_4/1(dout) -> ri_to_c23/2(im)
  conv_of_3/1(dout) -> ri_to_c23/1(re)
  ri_to_c01/1(c) -> a+bw/1
  conv_of_2/1(dout) -> ri_to_c01/2(im)
  conv_of_1/1(dout) -> ri_to_c01/1(re)
  Logical/1 -> of/1
  conv_of_4/2(of) -> Logical/4
  conv_of_3/2(of) -> Logical/3
  conv_of_2/2(of) -> Logical/2
  conv_of_1/2(of) -> Logical/1
  scale_4/1 -> conv_of_4/1(din)
  arith/4(a-bw_im) -> scale_4/1
  scale_3/1 -> conv_of_3/1(din)
  arith/3(a-bw_re) -> scale_3/1
  scale_2/1 -> conv_of_2/1(din)
  arith/2(a+bw_im) -> scale_2/1
  scale_1/1 -> conv_of_1/1(din)
  arith/1(a+bw_re) -> scale_1/1
  shift/1 -> Terminator/1
  sync/1 -> arith/3(sync)
  b/1 -> arith/2(b)
  a/1 -> arith/1(a)

== system xb_fft_32pt_core/fft_wideband_real1/fft_unscrambler/reorder1 ==
  sync : Inport
  en : Inport  Port=2
  din0 : Inport  Port=3
  din1 : Inport  Port=4
  Counter : xbsIndex_r4/Counter  cnt_type=Count Limited  cnt_to=23  operation=Up  start_count=0  cnt_by_val=1  arith_type=Unsigned  n_bits=5  bin_pt=0  load_pin=off  rst=on  en=on  explicit_period=on  period=1  dbl_ovrd=off  use_behavioral_HDL=off  implementation=Fabric  block_type=counter
  Mux : xbsIndex_r4/Mux  inputs=3  en=off  latency=1  precision=Full  arith_type=Unsigned  n_bits=16  bin_pt=14  quantization=Truncate  overflow=Wrap  dbl_ovrd=off  block_type=mux
  Slice1 : xbsIndex_r4/Slice  nbits=2  boolean_output=off  mode=Upper Bit Location + Width  bit1=0  base1=MSB of Input  bit0=0  base0=LSB of Input  dbl_ovrd=off  block_type=slice
  Slice2 : xbsIndex_r4/Slice  nbits=3  boolean_output=off  mode=Lower Bit Location + Width  bit1=0  base1=MSB of Input  bit0=0  base0=LSB of Input  dbl_ovrd=off  block_type=slice
  bram0 : xbsIndex_r4/Single Port RAM  depth=8  initVector=sin(pi*(0:15)/16)  distributed_mem=Block RAM  write_mode=Read Before Write  rst=off  init_reg=0  en=off  latency=2  dbl_ovrd=off  optimize=Area  use_rpm=on  block_type=spram
  bram1 : xbsIndex_r4/Single Port RAM  depth=8  initVector=sin(pi*(0:15)/16)  distributed_mem=Block RAM  write_mode=Read Before Write  rst=off  init_reg=0  en=off  latency=2  dbl_ovrd=off  optimize=Area  use_rpm=on  block_type=spram
  delay_d0 : xbsIndex_r4/Delay  rst=off  infoeditControl=Selection of Reset will increase slice count due to use of real FFs and instead of SRLs  en=off  latency=2  dbl_ovrd=off  reg_retiming=off  block_type=delay
  delay_din0 : xbsIndex_r4/Delay  rst=off  infoeditControl=Selection of Reset will increase slice count due to use of real FFs and instead of SRLs  en=off  latency=3  dbl_ovrd=off  reg_retiming=off  block_type=delay
  delay_din1 : xbsIndex_r4/Delay  rst=off  infoeditControl=Selection of Reset will increase slice count due to use of real FFs and instead of SRLs  en=off  latency=3  dbl_ovrd=off  reg_retiming=off  block_type=delay
  delay_map1 : xbsIndex_r4/Delay  rst=off  infoeditControl=Selection of Reset will increase slice count due to use of real FFs and instead of SRLs  en=off  latency=1  dbl_ovrd=off  reg_retiming=off  block_type=delay
  delay_map2 : xbsIndex_r4/Delay  rst=off  infoeditControl=Selection of Reset will increase slice count due to use of real FFs and instead of SRLs  en=off  latency=0  dbl_ovrd=off  reg_retiming=off  block_type=delay
  delay_sel : xbsIndex_r4/Delay  rst=off  infoeditControl=Selection of Reset will increase slice count due to use of real FFs and instead of SRLs  en=off  latency=2  dbl_ovrd=off  reg_retiming=off  block_type=delay
  delay_valid : xbsIndex_r4/Delay  rst=off  infoeditControl=Selection of Reset will increase slice count due to use of real FFs and instead of SRLs  en=off  latency=3  dbl_ovrd=off  reg_retiming=off  block_type=delay
  delay_we : xbsIndex_r4/Delay  rst=off  infoeditControl=Selection of Reset will increase slice count due to use of real FFs and instead of SRLs  en=off  latency=2  dbl_ovrd=off  reg_retiming=off  block_type=delay
  map1 : xbsIndex_r4/ROM  depth=8  initVector=[0 2 4 6 1 3 5 7]  distributed_mem=Distributed memory  rst=off  init_reg=0  en=off  latency=1  gui_display_data_type=Fixed-point  arith_type=Unsigned  n_bits=3  bin_pt=0  preci_type=Single  exp_width=8  frac_width=24  dbl_ovrd=off  optimize=Area  use_rpm=on  block_type=sprom
  map2 : xbsIndex_r4/ROM  depth=8  initVector=[0 2 4 6 1 3 5 7]  distributed_mem=Distributed memory  rst=off  init_reg=0  en=off  latency=1  gui_display_data_type=Fixed-point  arith_type=Unsigned  n_bits=3  bin_pt=0  preci_type=Single  exp_width=8  frac_width=24  dbl_ovrd=off  optimize=Area  use_rpm=on  block_type=sprom
  post_sync_delay : xbsIndex_r4/Delay  rst=off  infoeditControl=Selection of Reset will increase slice count due to use of real FFs and instead of SRLs  en=off  latency=3  dbl_ovrd=off  reg_retiming=off  block_type=delay
  pre_sync_delay : xbsIndex_r4/Delay  rst=off  infoeditControl=Selection of Reset will increase slice count due to use of real FFs and instead of SRLs  en=off  latency=2  dbl_ovrd=off  reg_retiming=off  block_type=delay
  sync_delay_en : Subsystem
  sync_out : Outport
  valid : Outport  Port=2
  dout0 : Outport  Port=3
  dout1 : Outport  Port=4
  wires:
  sync/1 -> Counter/1, pre_sync_delay/1
  en/1 -> Counter/2, delay_we/1, sync_delay_en/2(en)
  delay_we/1 -> bram1/3, bram0/3, delay_valid/1
  Counter/1 -> Slice2/1, Slice1/1
  Slice2/1 -> map1/1, delay_d0/1
  Mux/1 -> bram1/1, bram0/1
  map1/1 -> map2/1, delay_map1/1
  delay_map2/1 -> Mux/4
  map2/1 -> delay_map2/1
  delay_map1/1 -> Mux/3
  bram1/1 -> dout1/1
  delay_din1/1 -> bram1/2
  din1/1 -> delay_din1/1
  bram0/1 -> dout0/1
  delay_din0/1 -> bram0/2
  din0/1 -> delay_din0/1
  delay_d0/1 -> Mux/2
  delay_sel/1 -> Mux/1
  Slice1/1 -> delay_sel/1
  delay_valid/1 -> valid/1
  post_sync_delay/1 -> sync_out/1
  sync_delay_en/1(Out) -> post_sync_delay/1
  pre_sync_delay/1 -> sync_delay_en/1(In)

== system xb_fft_32pt_core/fft_wideband_real1/fft_unscrambler/square_transposer1 ==
  sync : Inport
  In1 : Inport  Port=2
  In2 : Inport  Port=3
  Delayb1 : xbsIndex_r4/Delay  rst=off  infoeditControl=Selection of Reset will increase slice count due to use of real FFs and instead of SRLs  en=off  latency=1  dbl_ovrd=off  reg_retiming=off  block_type=delay
  Delayb2 : xbsIndex_r4/Delay  rst=off  infoeditControl=Selection of Reset will increase slice count due to use of real FFs and instead of SRLs  en=off  latency=0  dbl_ovrd=off  reg_retiming=off  block_type=delay
  Delayf1 : xbsIndex_r4/Delay  rst=off  infoeditControl=Selection of Reset will increase slice count due to use of real FFs and instead of SRLs  en=off  latency=0  dbl_ovrd=off  reg_retiming=off  block_type=delay
  Delayf2 : xbsIndex_r4/Delay  rst=off  infoeditControl=Selection of Reset will increase slice count due to use of real FFs and instead of SRLs  en=off  latency=1  dbl_ovrd=off  reg_retiming=off  block_type=delay
  barrel_switcher : Subsystem
      settings: AttributesFormatString=n_inputs=1
  counter : xbsIndex_r4/Counter  cnt_type=Free Running  cnt_to=Inf  operation=Down  start_count=0  cnt_by_val=1  arith_type=Unsigned  n_bits=1  bin_pt=0  load_pin=off  rst=on  en=off  explicit_period=off  period=1  dbl_ovrd=off  use_behavioral_HDL=off  implementation=Fabric  use_rpm=on  block_type=counter
  delay0 : xbsIndex_r4/Delay  rst=off  infoeditControl=Selection of Reset will increase slice count due to use of real FFs and instead of SRLs  en=off  latency=1  dbl_ovrd=off  reg_retiming=off  block_type=delay
  sync_out : Outport
  Out1 : Outport  Port=2
  Out2 : Outport  Port=3
  wires:
  sync/1 -> barrel_switcher/2(sync_in), counter/1
  barrel_switcher/3(Out2) -> Delayb2/1  "barrel_switcher_Out2"
  barrel_switcher/2(Out1) -> Delayb1/1  "barrel_switcher_Out1"
  barrel_switcher/1(sync_out) -> delay0/1
  Delayf2/1 -> barrel_switcher/4(In2)  "barrel_switcher_In2"
  Delayf1/1 -> barrel_switcher/3(In1)  "barrel_switcher_In1"
  counter/1 -> barrel_switcher/1(sel)
  delay0/1 -> sync_out/1
  Delayb2/1 -> Out2/1
  In2/1 -> Delayf2/1
  Delayb1/1 -> Out1/1
  In1/1 -> Delayf1/1

== system xb_fft_32pt_core/fft_wideband_real1/fft_biplex_real_4x0/bi_real_unscr_4x/delay_srl0 ==
  in : Inport
  delay_ff : xbsIndex_r4/Delay  rst=off  infoeditControl=Selection of Reset will increase slice count due to use of real FFs and instead of SRLs  en=off  latency=1  dbl_ovrd=off  reg_retiming=off  block_type=delay
  delay_srl : xbsIndex_r4/Delay  rst=off  infoeditControl=Selection of Reset will increase slice count due to use of real FFs and instead of SRLs  en=off  latency=3  dbl_ovrd=off  reg_retiming=off  block_type=delay
  out : Outport
  wires:
  delay_srl/1 -> out/1
  delay_ff/1 -> delay_srl/1
  in/1 -> delay_ff/1

== system xb_fft_32pt_core/fft_wideband_real1/fft_biplex_real_4x0/bi_real_unscr_4x/delay_srl1 ==
  in : Inport
  delay_ff : xbsIndex_r4/Delay  rst=off  infoeditControl=Selection of Reset will increase slice count due to use of real FFs and instead of SRLs  en=off  latency=1  dbl_ovrd=off  reg_retiming=off  block_type=delay
  delay_srl : xbsIndex_r4/Delay  rst=off  infoeditControl=Selection of Reset will increase slice count due to use of real FFs and instead of SRLs  en=off  latency=3  dbl_ovrd=off  reg_retiming=off  block_type=delay
  out : Outport
  wires:
  delay_srl/1 -> out/1
  delay_ff/1 -> delay_srl/1
  in/1 -> delay_ff/1
